simulink model "CommSys_300_Bus_Area1_Part1"  (Simulink 8.0)
settings: Solver=ode45  StartTime=0.0  StopTime=3800  RelTol=1e-3
libraries: PiccSIM x82
settings Model: Creator=svenda  LastModifiedBy=svenda

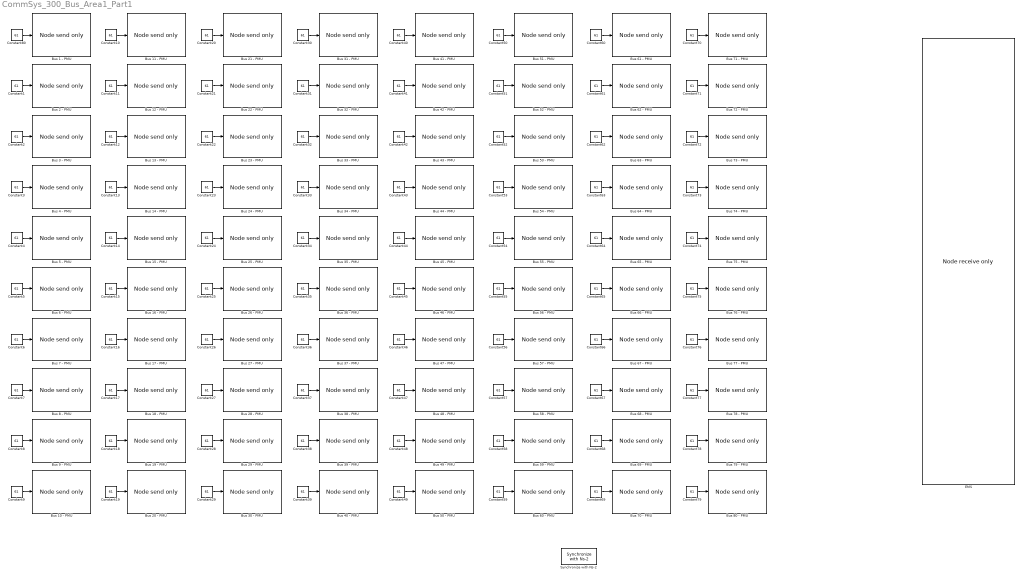
== system CommSys_300_Bus_Area1_Part1 ==
  Bus 1 - PMU : PiccSIM/Node send only  ID=0  time_or_seq=Timestamp  sendSchedule=Fixed sampling time  h=2  duty_cycle=1  sendEnable=off  pTypesSend=[10]  sendDataStructure={{'double'}}  externalID=off  sendID={[80]}  coordinates=[0, 0]  IP=NS2_IP
  Bus 10 - PMU : PiccSIM/Node send only  ID=9  time_or_seq=Timestamp  sendSchedule=Fixed sampling time  h=2  duty_cycle=1  sendEnable=off  pTypesSend=[19]  sendDataStructure={{'double'}}  externalID=off  sendID={[80]}  coordinates=[0, 0]  IP=NS2_IP
  Bus 11 - PMU : PiccSIM/Node send only  ID=10  time_or_seq=Timestamp  sendSchedule=Fixed sampling time  h=2  duty_cycle=1  sendEnable=off  pTypesSend=[110]  sendDataStructure={{'double'}}  externalID=off  sendID={[80]}  coordinates=[0, 0]  IP=NS2_IP
  Bus 12 - PMU : PiccSIM/Node send only  ID=11  time_or_seq=Timestamp  sendSchedule=Fixed sampling time  h=2  duty_cycle=1  sendEnable=off  pTypesSend=[111]  sendDataStructure={{'double'}}  externalID=off  sendID={[80]}  coordinates=[0, 0]  IP=NS2_IP
  Bus 13 - PMU : PiccSIM/Node send only  ID=12  time_or_seq=Timestamp  sendSchedule=Fixed sampling time  h=2  duty_cycle=1  sendEnable=off  pTypesSend=[112]  sendDataStructure={{'double'}}  externalID=off  sendID={[80]}  coordinates=[0, 0]  IP=NS2_IP
  Bus 14 - PMU : PiccSIM/Node send only  ID=13  time_or_seq=Timestamp  sendSchedule=Fixed sampling time  h=2  duty_cycle=1  sendEnable=off  pTypesSend=[113]  sendDataStructure={{'double'}}  externalID=off  sendID={[80]}  coordinates=[0, 0]  IP=NS2_IP
  Bus 15 - PMU : PiccSIM/Node send only  ID=14  time_or_seq=Timestamp  sendSchedule=Fixed sampling time  h=2  duty_cycle=1  sendEnable=off  pTypesSend=[114]  sendDataStructure={{'double'}}  externalID=off  sendID={[80]}  coordinates=[0, 0]  IP=NS2_IP
  Bus 16 - PMU : PiccSIM/Node send only  ID=15  time_or_seq=Timestamp  sendSchedule=Fixed sampling time  h=2  duty_cycle=1  sendEnable=off  pTypesSend=[115]  sendDataStructure={{'double'}}  externalID=off  sendID={[80]}  coordinates=[0, 0]  IP=NS2_IP
  Bus 17 - PMU : PiccSIM/Node send only  ID=16  time_or_seq=Timestamp  sendSchedule=Fixed sampling time  h=2  duty_cycle=1  sendEnable=off  pTypesSend=[116]  sendDataStructure={{'double'}}  externalID=off  sendID={[80]}  coordinates=[0, 0]  IP=NS2_IP
  Bus 18 - PMU : PiccSIM/Node send only  ID=17  time_or_seq=Timestamp  sendSchedule=Fixed sampling time  h=2  duty_cycle=1  sendEnable=off  pTypesSend=[117]  sendDataStructure={{'double'}}  externalID=off  sendID={[80]}  coordinates=[0, 0]  IP=NS2_IP
  Bus 19 - PMU : PiccSIM/Node send only  ID=18  time_or_seq=Timestamp  sendSchedule=Fixed sampling time  h=2  duty_cycle=1  sendEnable=off  pTypesSend=[118]  sendDataStructure={{'double'}}  externalID=off  sendID={[80]}  coordinates=[0, 0]  IP=NS2_IP
  Bus 2 - PMU : PiccSIM/Node send only  ID=1  time_or_seq=Timestamp  sendSchedule=Fixed sampling time  h=2  duty_cycle=1  sendEnable=off  pTypesSend=[11]  sendDataStructure={{'double'}}  externalID=off  sendID={[80]}  coordinates=[0, 0]  IP=NS2_IP
  Bus 20 - PMU : PiccSIM/Node send only  ID=19  time_or_seq=Timestamp  sendSchedule=Fixed sampling time  h=2  duty_cycle=1  sendEnable=off  pTypesSend=[119]  sendDataStructure={{'double'}}  externalID=off  sendID={[80]}  coordinates=[0, 0]  IP=NS2_IP
  Bus 21 - PMU : PiccSIM/Node send only  ID=20  time_or_seq=Timestamp  sendSchedule=Fixed sampling time  h=2  duty_cycle=1  sendEnable=off  pTypesSend=[120]  sendDataStructure={{'double'}}  externalID=off  sendID={[80]}  coordinates=[0, 0]  IP=NS2_IP
  Bus 22 - PMU : PiccSIM/Node send only  ID=21  time_or_seq=Timestamp  sendSchedule=Fixed sampling time  h=2  duty_cycle=1  sendEnable=off  pTypesSend=[121]  sendDataStructure={{'double'}}  externalID=off  sendID={[80]}  coordinates=[0, 0]  IP=NS2_IP
  Bus 23 - PMU : PiccSIM/Node send only  ID=22  time_or_seq=Timestamp  sendSchedule=Fixed sampling time  h=2  duty_cycle=1  sendEnable=off  pTypesSend=[122]  sendDataStructure={{'double'}}  externalID=off  sendID={[80]}  coordinates=[0, 0]  IP=NS2_IP
  Bus 24 - PMU : PiccSIM/Node send only  ID=23  time_or_seq=Timestamp  sendSchedule=Fixed sampling time  h=2  duty_cycle=1  sendEnable=off  pTypesSend=[123]  sendDataStructure={{'double'}}  externalID=off  sendID={[80]}  coordinates=[0, 0]  IP=NS2_IP
  Bus 25 - PMU : PiccSIM/Node send only  ID=24  time_or_seq=Timestamp  sendSchedule=Fixed sampling time  h=2  duty_cycle=1  sendEnable=off  pTypesSend=[124]  sendDataStructure={{'double'}}  externalID=off  sendID={[80]}  coordinates=[0, 0]  IP=NS2_IP
  Bus 26 - PMU : PiccSIM/Node send only  ID=25  time_or_seq=Timestamp  sendSchedule=Fixed sampling time  h=2  duty_cycle=1  sendEnable=off  pTypesSend=[125]  sendDataStructure={{'double'}}  externalID=off  sendID={[80]}  coordinates=[0, 0]  IP=NS2_IP
  Bus 27 - PMU : PiccSIM/Node send only  ID=26  time_or_seq=Timestamp  sendSchedule=Fixed sampling time  h=2  duty_cycle=1  sendEnable=off  pTypesSend=[126]  sendDataStructure={{'double'}}  externalID=off  sendID={[80]}  coordinates=[0, 0]  IP=NS2_IP
  Bus 28 - PMU : PiccSIM/Node send only  ID=27  time_or_seq=Timestamp  sendSchedule=Fixed sampling time  h=2  duty_cycle=1  sendEnable=off  pTypesSend=[127]  sendDataStructure={{'double'}}  externalID=off  sendID={[80]}  coordinates=[0, 0]  IP=NS2_IP
  Bus 29 - PMU : PiccSIM/Node send only  ID=28  time_or_seq=Timestamp  sendSchedule=Fixed sampling time  h=2  duty_cycle=1  sendEnable=off  pTypesSend=[128]  sendDataStructure={{'double'}}  externalID=off  sendID={[80]}  coordinates=[0, 0]  IP=NS2_IP
  Bus 3 - PMU : PiccSIM/Node send only  ID=2  time_or_seq=Timestamp  sendSchedule=Fixed sampling time  h=2  duty_cycle=1  sendEnable=off  pTypesSend=[12]  sendDataStructure={{'double'}}  externalID=off  sendID={[80]}  coordinates=[0, 0]  IP=NS2_IP
  Bus 30 - PMU : PiccSIM/Node send only  ID=29  time_or_seq=Timestamp  sendSchedule=Fixed sampling time  h=2  duty_cycle=1  sendEnable=off  pTypesSend=[129]  sendDataStructure={{'double'}}  externalID=off  sendID={[80]}  coordinates=[0, 0]  IP=NS2_IP
  Bus 31 - PMU : PiccSIM/Node send only  ID=30  time_or_seq=Timestamp  sendSchedule=Fixed sampling time  h=2  duty_cycle=1  sendEnable=off  pTypesSend=[130]  sendDataStructure={{'double'}}  externalID=off  sendID={[80]}  coordinates=[0, 0]  IP=NS2_IP
  Bus 32 - PMU : PiccSIM/Node send only  ID=31  time_or_seq=Timestamp  sendSchedule=Fixed sampling time  h=2  duty_cycle=1  sendEnable=off  pTypesSend=[131]  sendDataStructure={{'double'}}  externalID=off  sendID={[80]}  coordinates=[0, 0]  IP=NS2_IP
  Bus 33 - PMU : PiccSIM/Node send only  ID=32  time_or_seq=Timestamp  sendSchedule=Fixed sampling time  h=2  duty_cycle=1  sendEnable=off  pTypesSend=[132]  sendDataStructure={{'double'}}  externalID=off  sendID={[80]}  coordinates=[0, 0]  IP=NS2_IP
  Bus 34 - PMU : PiccSIM/Node send only  ID=33  time_or_seq=Timestamp  sendSchedule=Fixed sampling time  h=2  duty_cycle=1  sendEnable=off  pTypesSend=[133]  sendDataStructure={{'double'}}  externalID=off  sendID={[80]}  coordinates=[0, 0]  IP=NS2_IP
  Bus 35 - PMU : PiccSIM/Node send only  ID=34  time_or_seq=Timestamp  sendSchedule=Fixed sampling time  h=2  duty_cycle=1  sendEnable=off  pTypesSend=[134]  sendDataStructure={{'double'}}  externalID=off  sendID={[80]}  coordinates=[0, 0]  IP=NS2_IP
  Bus 36 - PMU : PiccSIM/Node send only  ID=35  time_or_seq=Timestamp  sendSchedule=Fixed sampling time  h=2  duty_cycle=1  sendEnable=off  pTypesSend=[135]  sendDataStructure={{'double'}}  externalID=off  sendID={[80]}  coordinates=[0, 0]  IP=NS2_IP
  Bus 37 - PMU : PiccSIM/Node send only  ID=36  time_or_seq=Timestamp  sendSchedule=Fixed sampling time  h=2  duty_cycle=1  sendEnable=off  pTypesSend=[136]  sendDataStructure={{'double'}}  externalID=off  sendID={[80]}  coordinates=[0, 0]  IP=NS2_IP
  Bus 38 - PMU : PiccSIM/Node send only  ID=37  time_or_seq=Timestamp  sendSchedule=Fixed sampling time  h=2  duty_cycle=1  sendEnable=off  pTypesSend=[137]  sendDataStructure={{'double'}}  externalID=off  sendID={[80]}  coordinates=[0, 0]  IP=NS2_IP
  Bus 39 - PMU : PiccSIM/Node send only  ID=38  time_or_seq=Timestamp  sendSchedule=Fixed sampling time  h=2  duty_cycle=1  sendEnable=off  pTypesSend=[138]  sendDataStructure={{'double'}}  externalID=off  sendID={[80]}  coordinates=[0, 0]  IP=NS2_IP
  Bus 4 - PMU : PiccSIM/Node send only  ID=3  time_or_seq=Timestamp  sendSchedule=Fixed sampling time  h=2  duty_cycle=1  sendEnable=off  pTypesSend=[13]  sendDataStructure={{'double'}}  externalID=off  sendID={[80]}  coordinates=[0, 0]  IP=NS2_IP
  Bus 40 - PMU : PiccSIM/Node send only  ID=39  time_or_seq=Timestamp  sendSchedule=Fixed sampling time  h=2  duty_cycle=1  sendEnable=off  pTypesSend=[139]  sendDataStructure={{'double'}}  externalID=off  sendID={[80]}  coordinates=[0, 0]  IP=NS2_IP
  Bus 41 - PMU : PiccSIM/Node send only  ID=40  time_or_seq=Timestamp  sendSchedule=Fixed sampling time  h=2  duty_cycle=1  sendEnable=off  pTypesSend=[140]  sendDataStructure={{'double'}}  externalID=off  sendID={[80]}  coordinates=[0, 0]  IP=NS2_IP
  Bus 42 - PMU : PiccSIM/Node send only  ID=41  time_or_seq=Timestamp  sendSchedule=Fixed sampling time  h=2  duty_cycle=1  sendEnable=off  pTypesSend=[141]  sendDataStructure={{'double'}}  externalID=off  sendID={[80]}  coordinates=[0, 0]  IP=NS2_IP
  Bus 43 - PMU : PiccSIM/Node send only  ID=42  time_or_seq=Timestamp  sendSchedule=Fixed sampling time  h=2  duty_cycle=1  sendEnable=off  pTypesSend=[142]  sendDataStructure={{'double'}}  externalID=off  sendID={[80]}  coordinates=[0, 0]  IP=NS2_IP
  Bus 44 - PMU : PiccSIM/Node send only  ID=43  time_or_seq=Timestamp  sendSchedule=Fixed sampling time  h=2  duty_cycle=1  sendEnable=off  pTypesSend=[143]  sendDataStructure={{'double'}}  externalID=off  sendID={[80]}  coordinates=[0, 0]  IP=NS2_IP
  Bus 45 - PMU : PiccSIM/Node send only  ID=44  time_or_seq=Timestamp  sendSchedule=Fixed sampling time  h=2  duty_cycle=1  sendEnable=off  pTypesSend=[144]  sendDataStructure={{'double'}}  externalID=off  sendID={[80]}  coordinates=[0, 0]  IP=NS2_IP
  Bus 46 - PMU : PiccSIM/Node send only  ID=45  time_or_seq=Timestamp  sendSchedule=Fixed sampling time  h=2  duty_cycle=1  sendEnable=off  pTypesSend=[145]  sendDataStructure={{'double'}}  externalID=off  sendID={[80]}  coordinates=[0, 0]  IP=NS2_IP
  Bus 47 - PMU : PiccSIM/Node send only  ID=46  time_or_seq=Timestamp  sendSchedule=Fixed sampling time  h=2  duty_cycle=1  sendEnable=off  pTypesSend=[146]  sendDataStructure={{'double'}}  externalID=off  sendID={[80]}  coordinates=[0, 0]  IP=NS2_IP
  Bus 48 - PMU : PiccSIM/Node send only  ID=47  time_or_seq=Timestamp  sendSchedule=Fixed sampling time  h=2  duty_cycle=1  sendEnable=off  pTypesSend=[147]  sendDataStructure={{'double'}}  externalID=off  sendID={[80]}  coordinates=[0, 0]  IP=NS2_IP
  Bus 49 - PMU : PiccSIM/Node send only  ID=48  time_or_seq=Timestamp  sendSchedule=Fixed sampling time  h=2  duty_cycle=1  sendEnable=off  pTypesSend=[148]  sendDataStructure={{'double'}}  externalID=off  sendID={[80]}  coordinates=[0, 0]  IP=NS2_IP
  Bus 5 - PMU : PiccSIM/Node send only  ID=4  time_or_seq=Timestamp  sendSchedule=Fixed sampling time  h=2  duty_cycle=1  sendEnable=off  pTypesSend=[14]  sendDataStructure={{'double'}}  externalID=off  sendID={[80]}  coordinates=[0, 0]  IP=NS2_IP
  Bus 50 - PMU : PiccSIM/Node send only  ID=49  time_or_seq=Timestamp  sendSchedule=Fixed sampling time  h=2  duty_cycle=1  sendEnable=off  pTypesSend=[149]  sendDataStructure={{'double'}}  externalID=off  sendID={[80]}  coordinates=[0, 0]  IP=NS2_IP
  Bus 51 - PMU : PiccSIM/Node send only  ID=50  time_or_seq=Timestamp  sendSchedule=Fixed sampling time  h=2  duty_cycle=1  sendEnable=off  pTypesSend=[150]  sendDataStructure={{'double'}}  externalID=off  sendID={[80]}  coordinates=[0, 0]  IP=NS2_IP
  Bus 52 - PMU : PiccSIM/Node send only  ID=51  time_or_seq=Timestamp  sendSchedule=Fixed sampling time  h=2  duty_cycle=1  sendEnable=off  pTypesSend=[151]  sendDataStructure={{'double'}}  externalID=off  sendID={[80]}  coordinates=[0, 0]  IP=NS2_IP
  Bus 53 - PMU : PiccSIM/Node send only  ID=52  time_or_seq=Timestamp  sendSchedule=Fixed sampling time  h=2  duty_cycle=1  sendEnable=off  pTypesSend=[152]  sendDataStructure={{'double'}}  externalID=off  sendID={[80]}  coordinates=[0, 0]  IP=NS2_IP
  Bus 54 - PMU : PiccSIM/Node send only  ID=53  time_or_seq=Timestamp  sendSchedule=Fixed sampling time  h=2  duty_cycle=1  sendEnable=off  pTypesSend=[153]  sendDataStructure={{'double'}}  externalID=off  sendID={[80]}  coordinates=[0, 0]  IP=NS2_IP
  Bus 55 - PMU : PiccSIM/Node send only  ID=54  time_or_seq=Timestamp  sendSchedule=Fixed sampling time  h=2  duty_cycle=1  sendEnable=off  pTypesSend=[154]  sendDataStructure={{'double'}}  externalID=off  sendID={[80]}  coordinates=[0, 0]  IP=NS2_IP
  Bus 56 - PMU : PiccSIM/Node send only  ID=55  time_or_seq=Timestamp  sendSchedule=Fixed sampling time  h=2  duty_cycle=1  sendEnable=off  pTypesSend=[155]  sendDataStructure={{'double'}}  externalID=off  sendID={[80]}  coordinates=[0, 0]  IP=NS2_IP
  Bus 57 - PMU : PiccSIM/Node send only  ID=56  time_or_seq=Timestamp  sendSchedule=Fixed sampling time  h=2  duty_cycle=1  sendEnable=off  pTypesSend=[156]  sendDataStructure={{'double'}}  externalID=off  sendID={[80]}  coordinates=[0, 0]  IP=NS2_IP
  Bus 58 - PMU : PiccSIM/Node send only  ID=57  time_or_seq=Timestamp  sendSchedule=Fixed sampling time  h=2  duty_cycle=1  sendEnable=off  pTypesSend=[157]  sendDataStructure={{'double'}}  externalID=off  sendID={[80]}  coordinates=[0, 0]  IP=NS2_IP
  Bus 59 - PMU : PiccSIM/Node send only  ID=58  time_or_seq=Timestamp  sendSchedule=Fixed sampling time  h=2  duty_cycle=1  sendEnable=off  pTypesSend=[158]  sendDataStructure={{'double'}}  externalID=off  sendID={[80]}  coordinates=[0, 0]  IP=NS2_IP
  Bus 6 - PMU : PiccSIM/Node send only  ID=5  time_or_seq=Timestamp  sendSchedule=Fixed sampling time  h=2  duty_cycle=1  sendEnable=off  pTypesSend=[15]  sendDataStructure={{'double'}}  externalID=off  sendID={[80]}  coordinates=[0, 0]  IP=NS2_IP
  Bus 60 - PMU : PiccSIM/Node send only  ID=59  time_or_seq=Timestamp  sendSchedule=Fixed sampling time  h=2  duty_cycle=1  sendEnable=off  pTypesSend=[159]  sendDataStructure={{'double'}}  externalID=off  sendID={[80]}  coordinates=[0, 0]  IP=NS2_IP
  Bus 61 - PMU : PiccSIM/Node send only  ID=60  time_or_seq=Timestamp  sendSchedule=Fixed sampling time  h=2  duty_cycle=1  sendEnable=off  pTypesSend=[160]  sendDataStructure={{'double'}}  externalID=off  sendID={[80]}  coordinates=[0, 0]  IP=NS2_IP
  Bus 62 - PMU : PiccSIM/Node send only  ID=61  time_or_seq=Timestamp  sendSchedule=Fixed sampling time  h=2  duty_cycle=1  sendEnable=off  pTypesSend=[161]  sendDataStructure={{'double'}}  externalID=off  sendID={[80]}  coordinates=[0, 0]  IP=NS2_IP
  Bus 63 - PMU : PiccSIM/Node send only  ID=62  time_or_seq=Timestamp  sendSchedule=Fixed sampling time  h=2  duty_cycle=1  sendEnable=off  pTypesSend=[162]  sendDataStructure={{'double'}}  externalID=off  sendID={[80]}  coordinates=[0, 0]  IP=NS2_IP
  Bus 64 - PMU : PiccSIM/Node send only  ID=63  time_or_seq=Timestamp  sendSchedule=Fixed sampling time  h=2  duty_cycle=1  sendEnable=off  pTypesSend=[163]  sendDataStructure={{'double'}}  externalID=off  sendID={[80]}  coordinates=[0, 0]  IP=NS2_IP
  Bus 65 - PMU : PiccSIM/Node send only  ID=64  time_or_seq=Timestamp  sendSchedule=Fixed sampling time  h=2  duty_cycle=1  sendEnable=off  pTypesSend=[164]  sendDataStructure={{'double'}}  externalID=off  sendID={[80]}  coordinates=[0, 0]  IP=NS2_IP
  Bus 66 - PMU : PiccSIM/Node send only  ID=65  time_or_seq=Timestamp  sendSchedule=Fixed sampling time  h=2  duty_cycle=1  sendEnable=off  pTypesSend=[165]  sendDataStructure={{'double'}}  externalID=off  sendID={[80]}  coordinates=[0, 0]  IP=NS2_IP
  Bus 67 - PMU : PiccSIM/Node send only  ID=66  time_or_seq=Timestamp  sendSchedule=Fixed sampling time  h=2  duty_cycle=1  sendEnable=off  pTypesSend=[166]  sendDataStructure={{'double'}}  externalID=off  sendID={[80]}  coordinates=[0, 0]  IP=NS2_IP
  Bus 68 - PMU : PiccSIM/Node send only  ID=67  time_or_seq=Timestamp  sendSchedule=Fixed sampling time  h=2  duty_cycle=1  sendEnable=off  pTypesSend=[167]  sendDataStructure={{'double'}}  externalID=off  sendID={[80]}  coordinates=[0, 0]  IP=NS2_IP
  Bus 69 - PMU : PiccSIM/Node send only  ID=68  time_or_seq=Timestamp  sendSchedule=Fixed sampling time  h=2  duty_cycle=1  sendEnable=off  pTypesSend=[168]  sendDataStructure={{'double'}}  externalID=off  sendID={[80]}  coordinates=[0, 0]  IP=NS2_IP
  Bus 7 - PMU : PiccSIM/Node send only  ID=6  time_or_seq=Timestamp  sendSchedule=Fixed sampling time  h=2  duty_cycle=1  sendEnable=off  pTypesSend=[16]  sendDataStructure={{'double'}}  externalID=off  sendID={[80]}  coordinates=[0, 0]  IP=NS2_IP
  Bus 70 - PMU : PiccSIM/Node send only  ID=69  time_or_seq=Timestamp  sendSchedule=Fixed sampling time  h=2  duty_cycle=1  sendEnable=off  pTypesSend=[169]  sendDataStructure={{'double'}}  externalID=off  sendID={[80]}  coordinates=[0, 0]  IP=NS2_IP
  Bus 71 - PMU : PiccSIM/Node send only  ID=70  time_or_seq=Timestamp  sendSchedule=Fixed sampling time  h=2  duty_cycle=1  sendEnable=off  pTypesSend=[170]  sendDataStructure={{'double'}}  externalID=off  sendID={[80]}  coordinates=[0, 0]  IP=NS2_IP
  Bus 72 - PMU : PiccSIM/Node send only  ID=71  time_or_seq=Timestamp  sendSchedule=Fixed sampling time  h=2  duty_cycle=1  sendEnable=off  pTypesSend=[171]  sendDataStructure={{'double'}}  externalID=off  sendID={[80]}  coordinates=[0, 0]  IP=NS2_IP
  Bus 73 - PMU : PiccSIM/Node send only  ID=72  time_or_seq=Timestamp  sendSchedule=Fixed sampling time  h=2  duty_cycle=1  sendEnable=off  pTypesSend=[172]  sendDataStructure={{'double'}}  externalID=off  sendID={[80]}  coordinates=[0, 0]  IP=NS2_IP
  Bus 74 - PMU : PiccSIM/Node send only  ID=73  time_or_seq=Timestamp  sendSchedule=Fixed sampling time  h=2  duty_cycle=1  sendEnable=off  pTypesSend=[173]  sendDataStructure={{'double'}}  externalID=off  sendID={[80]}  coordinates=[0, 0]  IP=NS2_IP
  Bus 75 - PMU : PiccSIM/Node send only  ID=74  time_or_seq=Timestamp  sendSchedule=Fixed sampling time  h=2  duty_cycle=1  sendEnable=off  pTypesSend=[174]  sendDataStructure={{'double'}}  externalID=off  sendID={[80]}  coordinates=[0, 0]  IP=NS2_IP
  Bus 76 - PMU : PiccSIM/Node send only  ID=75  time_or_seq=Timestamp  sendSchedule=Fixed sampling time  h=2  duty_cycle=1  sendEnable=off  pTypesSend=[175]  sendDataStructure={{'double'}}  externalID=off  sendID={[80]}  coordinates=[0, 0]  IP=NS2_IP
  Bus 77 - PMU : PiccSIM/Node send only  ID=76  time_or_seq=Timestamp  sendSchedule=Fixed sampling time  h=2  duty_cycle=1  sendEnable=off  pTypesSend=[176]  sendDataStructure={{'double'}}  externalID=off  sendID={[80]}  coordinates=[0, 0]  IP=NS2_IP
  Bus 78 - PMU : PiccSIM/Node send only  ID=77  time_or_seq=Timestamp  sendSchedule=Fixed sampling time  h=2  duty_cycle=1  sendEnable=off  pTypesSend=[177]  sendDataStructure={{'double'}}  externalID=off  sendID={[80]}  coordinates=[0, 0]  IP=NS2_IP
  Bus 79 - PMU : PiccSIM/Node send only  ID=78  time_or_seq=Timestamp  sendSchedule=Fixed sampling time  h=2  duty_cycle=1  sendEnable=off  pTypesSend=[178]  sendDataStructure={{'double'}}  externalID=off  sendID={[80]}  coordinates=[0, 0]  IP=NS2_IP
  Bus 8 - PMU : PiccSIM/Node send only  ID=7  time_or_seq=Timestamp  sendSchedule=Fixed sampling time  h=2  duty_cycle=1  sendEnable=off  pTypesSend=[17]  sendDataStructure={{'double'}}  externalID=off  sendID={[80]}  coordinates=[0, 0]  IP=NS2_IP
  Bus 80 - PMU : PiccSIM/Node send only  ID=79  time_or_seq=Timestamp  sendSchedule=Fixed sampling time  h=2  duty_cycle=1  sendEnable=off  pTypesSend=[179]  sendDataStructure={{'double'}}  externalID=off  sendID={[80]}  coordinates=[0, 0]  IP=NS2_IP
  Bus 9 - PMU : PiccSIM/Node send only  ID=8  time_or_seq=Timestamp  sendSchedule=Fixed sampling time  h=2  duty_cycle=1  sendEnable=off  pTypesSend=[18]  sendDataStructure={{'double'}}  externalID=off  sendID={[80]}  coordinates=[0, 0]  IP=NS2_IP
  Constant{1..80} (80 alike) : Constant  Value=61
  EMS : PiccSIM/Node receive only  ID=80  pTypes=[10, 11, 12, 13, 14, 15, 16, 17, 18, 19, 110, 111, 112, 113, 114, 115, 116, 117, 118, 119, 120, 121, 122, 123, 124, 125, 126, 127, 128, 129, 130, 131, 132, 133, 134, 135, 136, 137, 138, 139, 140, 141, 142, 143, 144, 145, 146, 147, 148, 149, 150, 151, 152, 153, 154, 155, 156, 157, 158, 159, 160, 161, 162, 163, 164, 165, 166, 167, 168, 169, 170, 171, 172, 173, 174, 175, 176, 177, 178, 179]  receiveDataLengths={{[1]}, {[1]}, {[1]}, {[1]}, {[1]}, {[1]}, {[1]}, {[1]}, {[1]}, {[1]},{[1]}, {[1]}, {[1]}, {[1]}, {[1]}, {[1]}, {[1]}, {[1]}, {[1]}, {[1]},{[1]}, {[1]}, {[1]}, {[1]}, {[1]}, {[1]}, {[1]}, {[1]}, {[1]}, {[1]},{[1]}, {[1]}, {[1]}, {[1]}, {[1]}, {[1]}, {[1]}, {[1]}, {[1]}, {[1]},{[1]}, {[1]}, {[1]}, {[1]}, {[1]}, {[1]}, {[1]}, {[1]}, {[1]}, {[1]},{[1]}, {[1]}, {[1]}, {[1]}, {[1]}, {[1]}, {[1]}, {[1]}, {[1]}, {[1]},{[1]}, {[1]}, {[1]}, {[1]}, {[1]}, {[1]}, {[1]}, {[1]}, {[1]}, {[1]},{[1]}, {[1]}, {[1]}, {[1]}, {[1]}, {[1]}, {[1]}, {[1]}, {[1]}, {[1]}}  receiveDataStructure={{'double'}, {'double'}, {'double'}, {'double'}, {'double'}, {'double'}, {'double'}, {'double'}, {'double'}, {'double'},{'double'}, {'double'}, {'double'}, {'double'}, {'double'}, {'double'}, {'double'}, {'double'}, {'double'}, {'double'},{'double'}, {'double'}, {'double'}, {'double'}, {'double'}, {'double'}, {'double'}, {'double'}, {'double'}, {'double'},{'double'}, {'double'}, {'double'}, {'double'}, {'double'}, {'double'}, {'double'}, {'double'}, {'double'}, {'double'},{'double'}, {'double'}, {'double'}, {'double'}, {'double'}, {'double'}, {'double'}, {'double'}, {'double'}, {'double'},{'double'}, {'double'}, {'double'}, {'double'}, {'double'}, {'double'}, {'double'}, {'double'}, {'double'}, {'double'},{'double'}, {'double'}, {'double'}, {'double'}, {'double'}, {'double'}, {'double'}, {'double'}, {'double'}, {'double'},{'double'}, {'double'}, {'double'}, {'double'}, {'double'}, {'double'}, {'double'}, {'double'}, {'double'}, {'double'}}  recFrom={[0], [1], [2], [3], [4], [5], [6], [7], [8], [9], [10], [11], [12], [13], [14], [15], [16], [17], [18], [19], [20], [21], [22], [23], [24], [25], [26], [27], [28], [29], [30], [31], [32], [33], [34], [35], [36], [37], [38], [39], [40], [41], [42], [43], [44], [45], [46], [47], [48], [49], [50], [51], [52], [53], [54], [55], [56], [57], [58], [59], [60], [61], [62], [63], [64], [65], [66], [67], [68], [69], [70], [71], [72], [73], [74], [75], [76], [77], [78], [79]}  coordinates=[0, 0]  IP=NS2_IP
  Synchronize with Ns-2 : PiccSIM/Synchronize with Ns-2  Priority=100000  c=1  port=23201  IP=NS2_IP
  wires:
  Constant1/1 -> Bus 2 - PMU/1
  Constant2/1 -> Bus 3 - PMU/1
  Constant3/1 -> Bus 4 - PMU/1
  Constant4/1 -> Bus 5 - PMU/1
  Constant5/1 -> Bus 6 - PMU/1
  Constant6/1 -> Bus 7 - PMU/1
  Constant7/1 -> Bus 8 - PMU/1
  Constant8/1 -> Bus 9 - PMU/1
  Constant9/1 -> Bus 10 - PMU/1
  Constant10/1 -> Bus 11 - PMU/1
  Constant11/1 -> Bus 12 - PMU/1
  Constant12/1 -> Bus 13 - PMU/1
  Constant13/1 -> Bus 14 - PMU/1
  Constant14/1 -> Bus 15 - PMU/1
  Constant15/1 -> Bus 16 - PMU/1
  Constant16/1 -> Bus 17 - PMU/1
  Constant17/1 -> Bus 18 - PMU/1
  Constant18/1 -> Bus 19 - PMU/1
  Constant19/1 -> Bus 20 - PMU/1
  Constant20/1 -> Bus 21 - PMU/1
  Constant21/1 -> Bus 22 - PMU/1
  Constant22/1 -> Bus 23 - PMU/1
  Constant23/1 -> Bus 24 - PMU/1
  Constant24/1 -> Bus 25 - PMU/1
  Constant25/1 -> Bus 26 - PMU/1
  Constant26/1 -> Bus 27 - PMU/1
  Constant27/1 -> Bus 28 - PMU/1
  Constant28/1 -> Bus 29 - PMU/1
  Constant29/1 -> Bus 30 - PMU/1
  Constant30/1 -> Bus 31 - PMU/1
  Constant31/1 -> Bus 32 - PMU/1
  Constant32/1 -> Bus 33 - PMU/1
  Constant33/1 -> Bus 34 - PMU/1
  Constant34/1 -> Bus 35 - PMU/1
  Constant35/1 -> Bus 36 - PMU/1
  Constant36/1 -> Bus 37 - PMU/1
  Constant37/1 -> Bus 38 - PMU/1
  Constant38/1 -> Bus 39 - PMU/1
  Constant39/1 -> Bus 40 - PMU/1
  Constant40/1 -> Bus 41 - PMU/1
  Constant41/1 -> Bus 42 - PMU/1
  Constant42/1 -> Bus 43 - PMU/1
  Constant43/1 -> Bus 44 - PMU/1
  Constant44/1 -> Bus 45 - PMU/1
  Constant45/1 -> Bus 46 - PMU/1
  Constant46/1 -> Bus 47 - PMU/1
  Constant47/1 -> Bus 48 - PMU/1
  Constant48/1 -> Bus 49 - PMU/1
  Constant49/1 -> Bus 50 - PMU/1
  Constant50/1 -> Bus 51 - PMU/1
  Constant51/1 -> Bus 52 - PMU/1
  Constant52/1 -> Bus 53 - PMU/1
  Constant53/1 -> Bus 54 - PMU/1
  Constant54/1 -> Bus 55 - PMU/1
  Constant55/1 -> Bus 56 - PMU/1
  Constant56/1 -> Bus 57 - PMU/1
  Constant57/1 -> Bus 58 - PMU/1
  Constant58/1 -> Bus 59 - PMU/1
  Constant59/1 -> Bus 60 - PMU/1
  Constant60/1 -> Bus 61 - PMU/1
  Constant61/1 -> Bus 62 - PMU/1
  Constant62/1 -> Bus 63 - PMU/1
  Constant63/1 -> Bus 64 - PMU/1
  Constant64/1 -> Bus 65 - PMU/1
  Constant65/1 -> Bus 66 - PMU/1
  Constant66/1 -> Bus 67 - PMU/1
  Constant67/1 -> Bus 68 - PMU/1
  Constant68/1 -> Bus 69 - PMU/1
  Constant69/1 -> Bus 70 - PMU/1
  Constant70/1 -> Bus 71 - PMU/1
  Constant71/1 -> Bus 72 - PMU/1
  Constant72/1 -> Bus 73 - PMU/1
  Constant73/1 -> Bus 74 - PMU/1
  Constant74/1 -> Bus 75 - PMU/1
  Constant75/1 -> Bus 76 - PMU/1
  Constant76/1 -> Bus 77 - PMU/1
  Constant77/1 -> Bus 78 - PMU/1
  Constant78/1 -> Bus 79 - PMU/1
  Constant79/1 -> Bus 80 - PMU/1
  Constant80/1 -> Bus 1 - PMU/1
